simulink model "model_observer_down_controller"  (R2024a)
settings: Solver=FixedStepAuto  StartTime=0.0  StopTime=20.0  RelTol=1e-3
undefined symbols (not defined in the file): A, B, C, D, G, K, N, Q, x0, x_hat0, Y
settings Model: Creator=anton  LastModifiedBy=anton

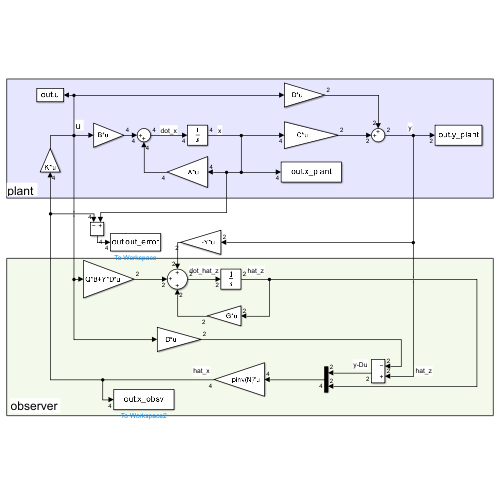
[thumbnail: Simulink's stored preview of the top-level diagram]
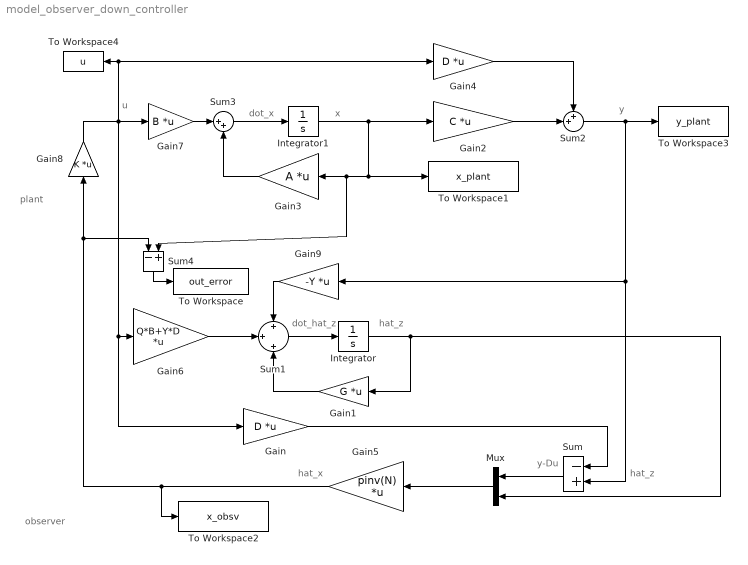
== system model_observer_down_controller ==
  note: y
  note: x
  note: dot_x
  note: u
  note: dot_hat_z
  note: hat_z
  note: hat_z
  note: y-Du
  note: hat_x
  note: observer
  note: plant
  Gain : Gain  Gain=D  Multiplication=Matrix(K*u)
  Gain1 : Gain  Gain=G  Multiplication=Matrix(K*u)
  Gain2 : Gain  Gain=C  Multiplication=Matrix(K*u)
  Gain3 : Gain  Gain=A  Multiplication=Matrix(K*u)
  Gain4 : Gain  Gain=D  Multiplication=Matrix(K*u)
  Gain5 : Gain  Gain=pinv(N)  Multiplication=Matrix(K*u)
  Gain6 : Gain  Gain=Q*B+Y*D  Multiplication=Matrix(K*u)
  Gain7 : Gain  Gain=B  Multiplication=Matrix(K*u)
  Gain8 : Gain  Gain=K  Multiplication=Matrix(K*u)
  Gain9 : Gain  Gain=-Y  Multiplication=Matrix(K*u)
  Integrator : Integrator  InitialCondition=x_hat0
  Integrator1 : Integrator  InitialCondition=x0
  Mux : Mux  Inputs=2
  Sum : Sum  Inputs=-+
  Sum1 : Sum  Inputs=+|+|+
  Sum2 : Sum  Inputs=++|
  Sum3 : Sum  Inputs=|++
  Sum4 : Sum  Inputs=-+
  To Workspace : ToWorkspace  VariableName=out_error  SaveFormat=Timeseries  SampleTime=-1
  To Workspace1 : ToWorkspace  VariableName=x_plant  SaveFormat=Timeseries  SampleTime=-1
  To Workspace2 : ToWorkspace  VariableName=x_obsv  SaveFormat=Timeseries  SampleTime=-1
  To Workspace3 : ToWorkspace  VariableName=y_plant  SaveFormat=Timeseries  SampleTime=-1
  To Workspace4 : ToWorkspace  VariableName=u  SaveFormat=Timeseries  SampleTime=-1
  wires:
  Integrator/1 -> Mux/2, Gain1/1
  Sum1/1 -> Integrator/1
  Sum3/1 -> Integrator1/1
  Gain3/1 -> Sum3/2
  Gain1/1 -> Sum1/3
  Gain/1 -> Sum/1
  Mux/1 -> Gain5/1
  Gain7/1 -> Sum3/1
  Gain8/1 -> Gain7/1, Gain/1, Gain6/1, Gain4/1, To Workspace4/1
  Gain5/1 -> Sum4/1, Gain8/1, To Workspace2/1
  Gain9/1 -> Sum1/1
  Sum/1 -> Mux/1
  Gain6/1 -> Sum1/2
  Gain4/1 -> Sum2/1
  Gain2/1 -> Sum2/2
  Sum2/1 -> Sum/2, Gain9/1, To Workspace3/1
  Integrator1/1 -> Gain2/1, Sum4/2, Gain3/1, To Workspace1/1
  Sum4/1 -> To Workspace/1
